simulink model "simulink_nonlineare_nonattrito_closedloop"  (R2025b)
settings: Solver=ode23  StartTime=0.0  StopTime=50  RelTol=1e-3
values from neighbouring files (symbols this model uses):
  alpha_0 = invpendulumP.alpha_0    [CODE_42_01.m]    (also in nonlinear_analisys_and_simulation.m)
  alpha_1 = invpendulumP.alpha_1    [CODE_42_01.m]    (also in nonlinear_analisys_and_simulation.m)
  g = invpendulumP.g    [CODE_42_01.m]    (also in nonlinear_analisys_and_simulation.m)
  I_0 = invpendulumP.I_0    [CODE_42_01.m]    (also in nonlinear_analisys_and_simulation.m)
  I_1 = invpendulumP.I_1    [CODE_42_01.m]    (also in nonlinear_analisys_and_simulation.m)
  I_2 = invpendulumP.I_2    [CODE_42_01.m]    (also in nonlinear_analisys_and_simulation.m)
  kd = 1    [CODE_42_01.m]    (also in nonlinear_analisys_and_simulation.m)
  kp = 8    [CODE_42_01.m]    (also in nonlinear_analisys_and_simulation.m)
  kt = invpendulumP.kt    [CODE_42_01.m]    (also in nonlinear_analisys_and_simulation.m)
  M = invpendulumP.M    [CODE_42_01.m]    (also in nonlinear_analisys_and_simulation.m)
  r = invpendulumP.r    [CODE_42_01.m]    (also in nonlinear_analisys_and_simulation.m)
settings Model: Creator=palla  LastModifiedBy=palla

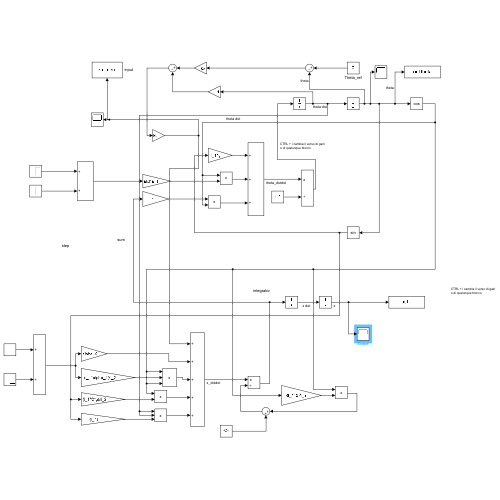
[thumbnail: Simulink's stored preview of the top-level diagram]
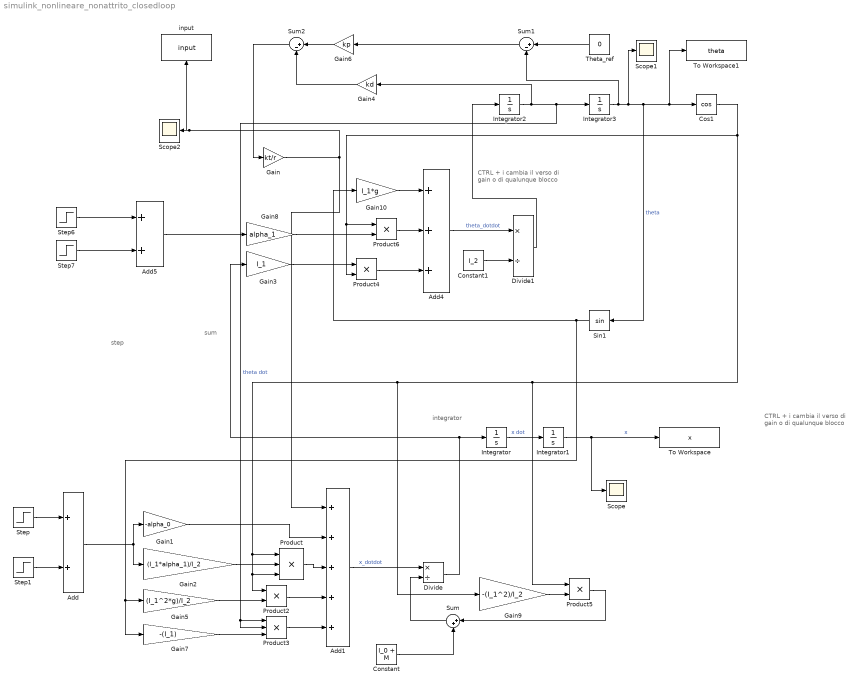
== system simulink_nonlineare_nonattrito_closedloop ==
  note: CTRL + i cambia il verso di gain
      | o di qualunque blocco
  note: sum
  note: integrator
  note: step
  note: CTRL + i cambia il verso di gain
      | o di qualunque blocco
  Add : Sum
  Add1 : Sum  Inputs=+++++
  Add4 : Sum  Inputs=+++
  Add5 : Sum
  Constant : Constant  Value=I_0 + M
  Constant1 : Constant  Value=I_2
  Cos1 : Trigonometry  Operator=cos
  Divide : Product  Inputs=*/
  Divide1 : Product  Inputs=*/
  Gain : Gain  Gain=kt/r
  Gain1 : Gain  Gain=-alpha_0
  Gain10 : Gain  Gain=I_1*g
  Gain2 : Gain  Gain=(I_1*alpha_1)/I_2
  Gain3 : Gain  Gain=I_1
  Gain4 : Gain  Gain=kd
  Gain5 : Gain  Gain=(I_1^2*g)/I_2
  Gain6 : Gain  Gain=kp
  Gain7 : Gain  Gain=-(I_1)
  Gain8 : Gain  Gain=alpha_1
  Gain9 : Gain  Gain=-(I_1^2)/I_2
  Integrator{,1..3} (4 alike) : Integrator
  Product : Product  Inputs=3
  Product{2,4..6} (4 alike) : Product
  Product3 : Product  Inputs=3
  Scope : Scope
      settings: ActiveDisplayYMinimum=-1  ActiveDisplayYMaximum=1
  Scope1 : Scope
      settings: ActiveDisplayYMinimum=-0.053191416890527685  ActiveDisplayYMaximum=0.062229691339195939
  Scope2 : Scope
      settings: ActiveDisplayYMinimum=-1  ActiveDisplayYMaximum=1  DataLoggingVariableName=ScopeData2
  Sin1 : Trigonometry
  Step : Step  SampleTime=0
  Step1 : Step  Time=3  After=-1  SampleTime=0
  Step6 : Step  SampleTime=0
  Step7 : Step  Time=3  After=-1  SampleTime=0
  Sum : Sum  Inputs=|++
  Sum1 : Sum  Inputs=|+-
  Sum2 : Sum  Inputs=|+-
  Theta_ref : Constant  Value=0
  To Workspace : ToWorkspace  VariableName=x  SampleTime=-1
  To Workspace1 : ToWorkspace  VariableName=theta  SampleTime=-1
  input : ToWorkspace  VariableName=input  SampleTime=-1
  wires:
  Divide/1 -> Gain3/1, Integrator/1
  Gain1/1 -> Add1/2
  Gain2/1 -> Product/2
  Product/1 -> Add1/3
  Gain9/1 -> Product5/2
  Step/1 -> Add/1
  Step7/1 -> Add5/2
  Gain7/1 -> Product3/3
  Integrator2/1 -> Gain4/1, Product3/1, Product3/2, Integrator3/1  "theta dot"
  Product2/1 -> Add1/4
  Constant/1 -> Sum/2
  Integrator/1 -> Integrator1/1  "x dot"
  Step6/1 -> Add5/1
  Product3/1 -> Add1/5
  Add4/1 -> Divide1/1  "theta_dotdot"
  Product6/1 -> Add4/2
  Product4/1 -> Add4/3
  Sin1/1 -> Gain10/1, Gain7/1, Gain5/1
  Product5/1 -> Sum/1
  Add1/1 -> Divide/1  "x_dotdot"
  Gain10/1 -> Add4/1
  Sum/1 -> Divide/2
  Integrator3/1 -> Sum1/2, To Workspace1/1, Cos1/1, Sin1/1, Scope1/1  "theta"
  Gain8/1 -> Product6/2
  Cos1/1 -> Product5/1, Gain9/1, Product/1, Product2/1, Product/3, Product4/2, Product6/1
  Add/1 -> Gain1/1, Gain2/1
  Gain3/1 -> Product4/1
  Step1/1 -> Add/2
  Divide1/1 -> Integrator2/1
  Add5/1 -> Gain8/1
  Integrator1/1 -> To Workspace/1, Scope/1  "x"
  Constant1/1 -> Divide1/2
  Theta_ref/1 -> Sum1/1
  Sum1/1 -> Gain6/1
  Gain6/1 -> Sum2/1
  Gain4/1 -> Sum2/2
  Sum2/1 -> Gain/1
  Gain/1 -> Add1/1, Scope2/1, input/1
  Gain5/1 -> Product2/2
